simulink model "HZNN_11612319_Ajay"  (R2021a)
settings: Solver=VariableStepAuto  StartTime=0.0  StopTime=1.0  RelTol=1e-8  AbsTol=1e-8
InitFcn:
  | k=10;
  | m=5;
  | I=eye(2);
libraries: neural x1
settings Model: Creator=Mannaiyar  LastModifiedBy=Mannaiyar
settings SolverCC: ZeroCrossControl=DisableAll

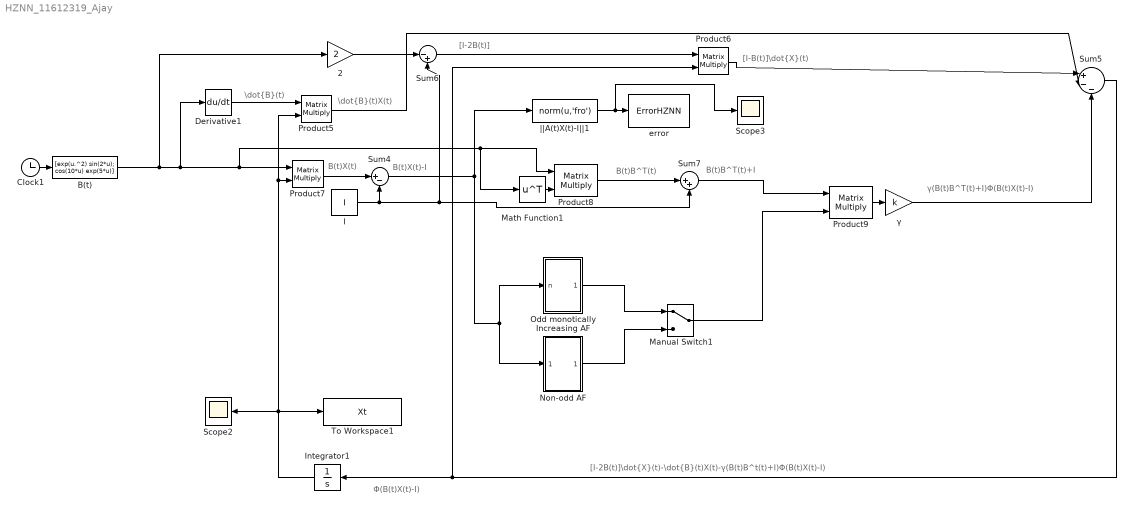
== system HZNN_11612319_Ajay ==
  note: Φ(B(t)X(t)-I)
  note: B(t)X(t)
  note: \dot{B}(t)X(t)
  note: \dot{B}(t)
  note: B(t)B^T(t)
  note: B(t)X(t)-I
  note: [I-2B(t)]
  note: [I-B(t)]\dot{X}(t)
  note: [I-2B(t)]\dot{X}(t)-\dot{B}(t)X(t)-γ(B(t)B^t(t)+I)Φ(B(t)X(t)-I)
  note: B(t)B^T(t)+I
  note: γ(B(t)B^T(t)+I)Φ(B(t)X(t)-I)
  2 : Gain  Gain=2
  B(t) : MATLABFcn  MATLABFcn=[exp(u.^2) sin(2*u); cos(10*u) exp(5*u)]  Output1D=off
  Clock1 : Clock
  Derivative1 : Derivative
  Integrator1 : Integrator
  Manual Switch1 : ManualSwitch
  Math Function1 : Math  Operator=transpose  SignedPower=on  SaturateOnIntegerOverflow=on
  Non-odd AF : Subsystem
  Odd monotically Increasing AF : Subsystem
  Product{5..9} (5 alike) : Product  Multiplication=Matrix(*)
  Scope2 : Scope
  Scope3 : Scope
  Sum4 : Sum  Inputs=|+-
  Sum5 : Sum  Inputs=|+--
  Sum6 : Sum  Inputs=|-+
  Sum7 : Sum  Inputs=|++
  To Workspace1 : ToWorkspace  VariableName=Xt  SaveFormat=Timeseries  SampleTime=-1
  error : ToWorkspace  VariableName=ErrorHZNN  SaveFormat=Timeseries  SampleTime=-1
  ||A(t)X(t)-I||1 : MATLABFcn  MATLABFcn=norm(u,'fro')
  "Ι " : Constant  Value=I  VectorParams1D=off
  γ : Gain  Gain=k
  wires:
  Sum7/1 -> Product9/1
  Product9/1 -> γ/1
  Product8/1 -> Sum7/1
  2/1 -> Sum6/1
  Integrator1/1 -> Product5/2, Product7/2, Scope2/1, To Workspace1/1
  Manual Switch1/1 -> Product9/2
  Product6/1 -> Sum5/1
  Sum6/1 -> Product6/1
  Math Function1/1 -> Product8/2
  Derivative1/1 -> Product5/1
  "Ι "/1 -> Sum7/2, Sum6/2, Sum4/2
  Sum4/1 -> Odd monotically Increasing AF/1(n), Non-odd AF/1(In1), ||A(t)X(t)-I||1/1
  Product5/1 -> Sum5/2
  Odd monotically Increasing AF/1(Out1) -> Manual Switch1/1
  B(t)/1 -> Math Function1/1, Product8/1, Product7/1, Derivative1/1, 2/1
  Product7/1 -> Sum4/1
  Sum5/1 -> Integrator1/1, Product6/2
  γ/1 -> Sum5/3
  ||A(t)X(t)-I||1/1 -> Scope3/1, error/1
  Non-odd AF/1(Out1) -> Manual Switch1/2
  Clock1/1 -> B(t)/1

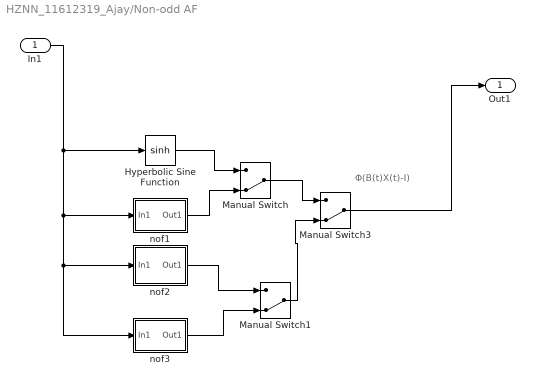
== system HZNN_11612319_Ajay/Non-odd AF ==
  note: Φ(B(t)X(t)-I)
  In1 : Inport
  Hyperbolic Sine Function : Trigonometry  Operator=sinh
  Manual Switch : ManualSwitch  CurrentSetting=0
  Manual Switch1 : ManualSwitch  CurrentSetting=0
  Manual Switch3 : ManualSwitch  CurrentSetting=0
  "nof1 " : Subsystem
  nof2 : Subsystem
  nof3 : Subsystem
  Out1 : Outport
  wires:
  Hyperbolic Sine Function/1 -> Manual Switch/1
  nof2/1(Out1) -> Manual Switch1/1
  In1/1 -> nof3/1(In1), nof2/1(In1), "nof1 "/1(In1), Hyperbolic Sine Function/1
  "nof1 "/1(Out1) -> Manual Switch/2
  Manual Switch/1 -> Manual Switch3/1
  Manual Switch1/1 -> Manual Switch3/2
  nof3/1(Out1) -> Manual Switch1/2
  Manual Switch3/1 -> Out1/1

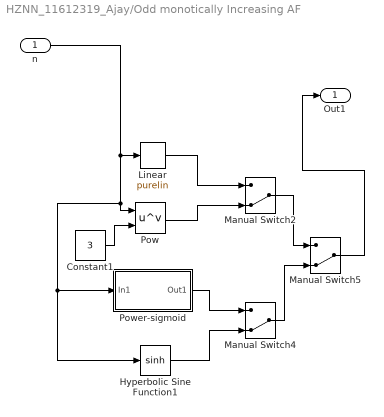
== system HZNN_11612319_Ajay/Odd monotically Increasing AF ==
  n : Inport
  Constant1 : Constant  Value=3
  Hyperbolic Sine Function1 : Trigonometry  Operator=sinh
  Linear : neural/Transfer Functions/purelin
  Manual Switch2 : ManualSwitch  CurrentSetting=0
  Manual Switch4 : ManualSwitch  CurrentSetting=0
  Manual Switch5 : ManualSwitch  CurrentSetting=0
  Pow : Math  Operator=pow  SignedPower=on  SaturateOnIntegerOverflow=on
  "Power-sigmoid " : Subsystem
  Out1 : Outport
  wires:
  Linear/1 -> Manual Switch2/1
  Hyperbolic Sine Function1/1 -> Manual Switch4/2
  Constant1/1 -> Pow/2
  Manual Switch2/1 -> Manual Switch5/1
  n/1 -> Hyperbolic Sine Function1/1, "Power-sigmoid "/1(In1), Pow/1, Linear/1
  "Power-sigmoid "/1(Out1) -> Manual Switch4/1
  Manual Switch4/1 -> Manual Switch5/2
  Pow/1 -> Manual Switch2/2
  Manual Switch5/1 -> Out1/1

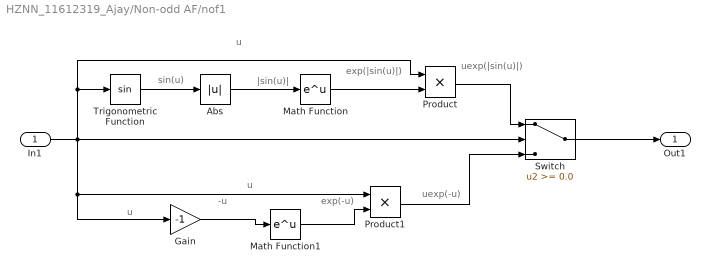
== system HZNN_11612319_Ajay/Non-odd AF/nof1  ==
  note: uexp(-u)
  note: exp(-u)
  note: -u
  note: u
  note: u
  note: u
  note: exp(|sin(u)|)
  note: |sin(u)|
  note: sin(u)
  note: uexp(|sin(u)|)
  In1 : Inport
  Abs : Abs
  Gain : Gain  Gain=-1
  Math Function : Math  SignedPower=on  SaturateOnIntegerOverflow=on
  Math Function1 : Math  SignedPower=on  SaturateOnIntegerOverflow=on
  Product : Product
  Product1 : Product
  Switch : Switch  Threshold=0.0
  Trigonometric Function : Trigonometry
  Out1 : Outport
  wires:
  Switch/1 -> Out1/1
  In1/1 -> Gain/1, Product1/1, Product/1, Trigonometric Function/1, Switch/2
  Trigonometric Function/1 -> Abs/1
  Abs/1 -> Math Function/1
  Product/1 -> Switch/1
  Product1/1 -> Switch/3
  Math Function1/1 -> Product1/2
  Gain/1 -> Math Function1/1
  Math Function/1 -> Product/2

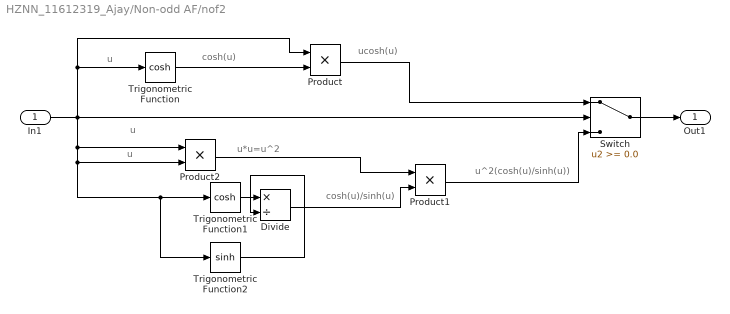
== system HZNN_11612319_Ajay/Non-odd AF/nof2 ==
  note: u^2(cosh(u)/sinh(u))
  note: cosh(u)/sinh(u)
  note: u*u=u^2
  note: u
  note: u
  note: ucosh(u)
  note: cosh(u)
  note: u
  In1 : Inport
  Divide : Product  Inputs=*/
  Product : Product
  Product1 : Product
  Product2 : Product
  Switch : Switch  Threshold=0.0
  Trigonometric Function : Trigonometry  Operator=cosh
  Trigonometric Function1 : Trigonometry  Operator=cosh
  Trigonometric Function2 : Trigonometry  Operator=sinh
  Out1 : Outport
  wires:
  Switch/1 -> Out1/1
  In1/1 -> Product2/1, Trigonometric Function2/1, Trigonometric Function1/1, Product2/2, Product/1, Trigonometric Function/1, Switch/2
  Product/1 -> Switch/1
  Product1/1 -> Switch/3
  Divide/1 -> Product1/2
  Trigonometric Function/1 -> Product/2
  Product2/1 -> Product1/1
  Trigonometric Function1/1 -> Divide/1
  Trigonometric Function2/1 -> Divide/2

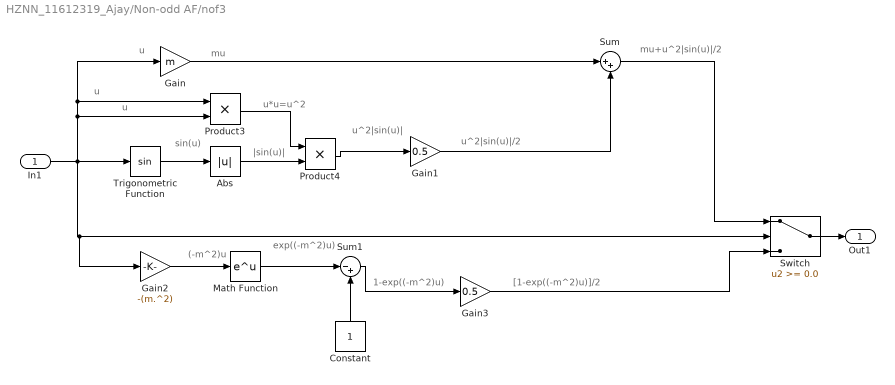
== system HZNN_11612319_Ajay/Non-odd AF/nof3 ==
  note: exp((-m^2)u)
  note: (-m^2)u
  note: mu+u^2|sin(u)|/2
  note: u^2|sin(u)|/2
  note: u^2|sin(u)|
  note: |sin(u)|
  note: sin(u)
  note: u*u=u^2
  note: u
  note: u
  note: mu
  note: u
  note: 1-exp((-m^2)u)
  note: [1-exp((-m^2)u)]/2
  In1 : Inport
  Abs : Abs
  Constant : Constant
  Gain : Gain  Gain=m
  Gain1 : Gain  Gain=0.5
  Gain2 : Gain  Gain=-(m.^2)
  Gain3 : Gain  Gain=0.5
  Math Function : Math  SignedPower=on  SaturateOnIntegerOverflow=on
  Product3 : Product
  Product4 : Product
  Sum : Sum  Inputs=|++
  Sum1 : Sum  Inputs=|-+
  Switch : Switch  Threshold=0.0
  Trigonometric Function : Trigonometry
  Out1 : Outport
  wires:
  Switch/1 -> Out1/1
  In1/1 -> Trigonometric Function/1, Gain2/1, Switch/2, Product3/2, Product3/1, Gain/1
  Trigonometric Function/1 -> Abs/1
  Abs/1 -> Product4/2
  Product3/1 -> Product4/1
  Product4/1 -> Gain1/1
  Gain1/1 -> Sum/2
  Gain/1 -> Sum/1
  Sum/1 -> Switch/1
  Gain2/1 -> Math Function/1
  Math Function/1 -> Sum1/1
  Constant/1 -> Sum1/2
  Sum1/1 -> Gain3/1
  Gain3/1 -> Switch/3

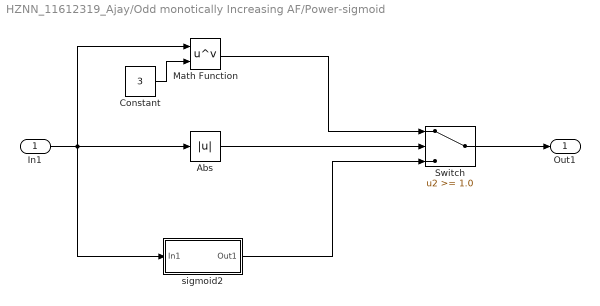
== system HZNN_11612319_Ajay/Odd monotically Increasing AF/Power-sigmoid  ==
  In1 : Inport
  Abs : Abs
  Constant : Constant  Value=3
  Math Function : Math  Operator=pow  SignedPower=on  SaturateOnIntegerOverflow=on
  Switch : Switch  Threshold=1.0
  "sigmoid2 " : Subsystem
  Out1 : Outport
  wires:
  Switch/1 -> Out1/1
  Abs/1 -> Switch/2
  "sigmoid2 "/1(Out1) -> Switch/3
  Constant/1 -> Math Function/2
  Math Function/1 -> Switch/1
  In1/1 -> "sigmoid2 "/1(In1), Math Function/1, Abs/1

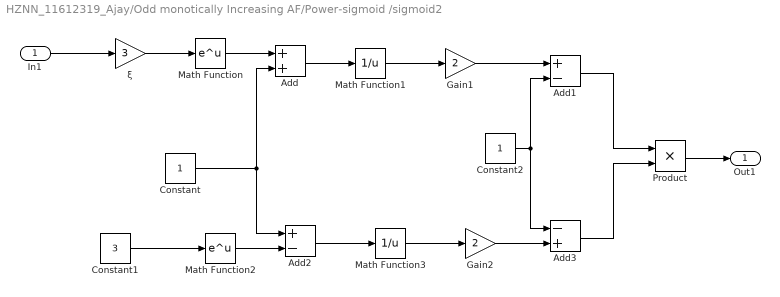
== system HZNN_11612319_Ajay/Odd monotically Increasing AF/Power-sigmoid /sigmoid2  ==
  In1 : Inport
  Add : Sum
  Add1 : Sum  Inputs=+-
  Add2 : Sum  Inputs=+-
  Add3 : Sum  Inputs=-+
  Constant : Constant
  Constant1 : Constant  Value=3
  Constant2 : Constant
  Gain1 : Gain  Gain=2
  Gain2 : Gain  Gain=2
  Math Function : Math  SignedPower=on  SaturateOnIntegerOverflow=on
  Math Function1 : Math  Operator=reciprocal  SignedPower=on  SaturateOnIntegerOverflow=on
  Math Function2 : Math  SignedPower=on  SaturateOnIntegerOverflow=on
  Math Function3 : Math  Operator=reciprocal  SignedPower=on  SaturateOnIntegerOverflow=on
  Product : Product  RndMeth=Zero
  ξ : Gain  Gain=3
  Out1 : Outport
  wires:
  ξ/1 -> Math Function/1
  In1/1 -> ξ/1
  Math Function1/1 -> Gain1/1
  Gain1/1 -> Add1/1
  Product/1 -> Out1/1
  Add1/1 -> Product/1
  Math Function/1 -> Add/1
  Add/1 -> Math Function1/1
  Constant1/1 -> Math Function2/1
  Math Function2/1 -> Add2/2
  Constant/1 -> Add2/1, Add/2
  Add2/1 -> Math Function3/1
  Math Function3/1 -> Gain2/1
  Constant2/1 -> Add3/1, Add1/2
  Gain2/1 -> Add3/2
  Add3/1 -> Product/2
